simulink model "Custom_mod"  (R2021a)
settings: configuration reference "AION_IDS_Speedgoat" (kept outside this file)
undefined symbols (not defined in the file): EPSILON
libraries: simulink x1
Description:
  | 自定义取模
settings Model: DataDictionary=Custom_Mod.sldd  Creator=xinrui  LastModifiedBy=Administrator
settings ConfigSetRef: SourceName=AION_IDS_Speedgoat

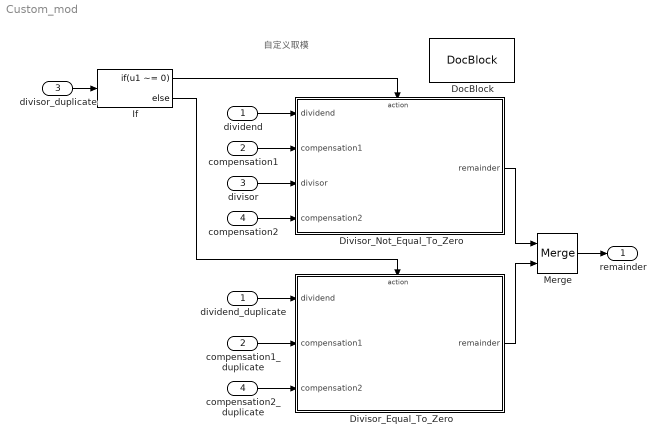
== system Custom_mod ==
  note: 自定义取模
  dividend : Inport  Description=被除数（待取模的数），实数，无量纲。  OutDataTypeStr=double  PortDimensions=1
  compensation1 : Inport  Description=用于调整取模前数值范围的补偿值1，实数，无量纲。  Port=2  OutDataTypeStr=double  PortDimensions=1
  divisor : Inport  Description=除数，实数，无量纲。  Port=3  OutDataTypeStr=double  PortDimensions=1
  compensation2 : Inport  Description=用于调整取模后数值范围的补偿值2，实数，无量纲。  Port=4  OutDataTypeStr=double  PortDimensions=1
  Divisor_Equal_To_Zero : Subsystem  Description=被除数等于0时直接输出被除数变换数值范围的结果。  TreatAsAtomicUnit=on
  Divisor_Not_Equal_To_Zero : Subsystem  Description=被除数不等于0时可依照公式计算余数，输出变换数值范围后的结果。  TreatAsAtomicUnit=on
  DocBlock : simulink/Model-Wide Utilities/DocBlock  DocumentType=HTML  mask(DocBlock){}
      mask Display:
      | plot([.8 0 0 1 1 .8 .8 1],[1 1 0 0 .8 1 .8 .8]);
      | text(.5,.6,'CHANGELOG','horizontalalignment','center');
      | text(.95,.05,get_param(gcb,'DocumentType'),'verticalalignment','bottom','horizontalalignment','right');
  If : If  IfExpression=u1 ~= 0
  Merge : Merge
  compensation1_duplicate : InportShadow  Description=用于调整取模前数值范围的补偿值1，实数，无量纲。  Port=2  OutDataTypeStr=double  PortDimensions=1
  compensation2_duplicate : InportShadow  Description=用于调整取模后数值范围的补偿值2，实数，无量纲。  Port=4  OutDataTypeStr=double  PortDimensions=1
  dividend_duplicate : InportShadow  Description=被除数（待取模的数），实数，无量纲。  OutDataTypeStr=double  PortDimensions=1
  divisor_duplicate : InportShadow  Description=除数，实数，无量纲。  Port=3  OutDataTypeStr=double  PortDimensions=1
  remainder : Outport  Description=余数，实数，无量纲。
  wires:
  dividend/1 -> Divisor_Not_Equal_To_Zero/1(dividend)
  compensation1/1 -> Divisor_Not_Equal_To_Zero/2(compensation1)
  divisor/1 -> Divisor_Not_Equal_To_Zero/3(divisor)
  compensation2/1 -> Divisor_Not_Equal_To_Zero/4(compensation2)
  divisor_duplicate/1 -> If/1
  If/1 -> Divisor_Not_Equal_To_Zero/Action
  Divisor_Not_Equal_To_Zero/1(remainder) -> Merge/1
  Divisor_Equal_To_Zero/1(remainder) -> Merge/2
  Merge/1 -> remainder/1
  compensation1_duplicate/1 -> Divisor_Equal_To_Zero/2(compensation1)
  compensation2_duplicate/1 -> Divisor_Equal_To_Zero/3(compensation2)
  dividend_duplicate/1 -> Divisor_Equal_To_Zero/1(dividend)
  If/2 -> Divisor_Equal_To_Zero/Action

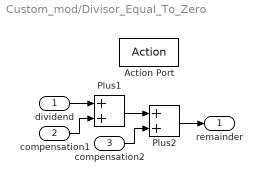
== system Custom_mod/Divisor_Equal_To_Zero ==
  dividend : Inport  Description=被除数（待取模的数），实数，无量纲。  OutDataTypeStr=double  PortDimensions=1
  compensation1 : Inport  Description=用于调整取模前数值范围的补偿值1，实数，无量纲。  Port=2  OutDataTypeStr=double  PortDimensions=1
  compensation2 : Inport  Description=用于调整取模后数值范围的补偿值2，实数，无量纲。  Port=3  OutDataTypeStr=double  PortDimensions=1
  Action Port : ActionPort  ActionPortLabel=else
  Plus1 : Sum  Description=将原始值通过补偿值1调整到指定数值范围区间。
  Plus2 : Sum  Description=将计算结果通过补偿值2调整到指定数值范围区间。
  remainder : Outport  Description=余数，实数，无量纲。
  wires:
  dividend/1 -> Plus1/1
  Plus2/1 -> remainder/1
  compensation2/1 -> Plus2/2
  Plus1/1 -> Plus2/1
  compensation1/1 -> Plus1/2

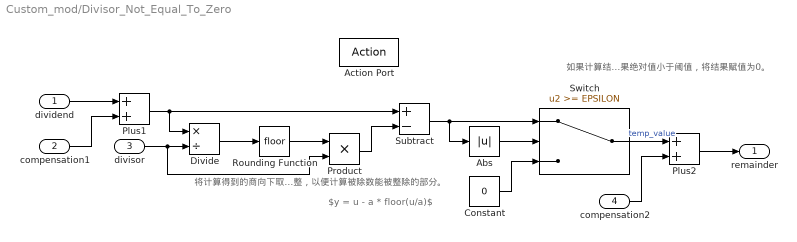
== system Custom_mod/Divisor_Not_Equal_To_Zero ==
  note: $y = u - a * floor(u/a)$
  note: 如果计算结果绝对值小于阈值，将结果赋值为0。
  note: 将计算得到的商向下取整，以便计算被除数能被整除的部分。
  dividend : Inport  Description=被除数（待取模的数），实数，无量纲。  OutDataTypeStr=double  PortDimensions=1
  compensation1 : Inport  Description=用于调整取模前数值范围的补偿值1，实数，无量纲。  Port=2  OutDataTypeStr=double  PortDimensions=1
  divisor : Inport  Description=除数，实数，无量纲。  Port=3  OutDataTypeStr=double  PortDimensions=1
  compensation2 : Inport  Description=用于调整取模后数值范围的补偿值2，实数，无量纲。  Port=4  OutDataTypeStr=double  PortDimensions=1
  Action Port : ActionPort  ActionPortLabel=if(u1 ~= 0)
  Abs : Abs
  Constant : Constant  Value=0  OutDataTypeStr=double  SampleTime=-1
  Divide : Product  Description=求被除数除以除数的商。  Inputs=*/
  Plus1 : Sum  Description=将原始值通过补偿值1调整到指定数值范围区间。
  Plus2 : Sum  Description=将计算结果通过补偿值2调整到指定数值范围区间。
  Product : Product  Description=将除数与整数形式的商相乘得到被除数能被整除部分
  Rounding Function : Rounding  Description=将计算得到的商向下取整，以便计算被除数能被整除的部分。
  Subtract : Sum  Description=将被除数减去能被整除部分，得到余数。  Inputs=+-
  Switch : Switch  Description=如果计算结果绝对值小于阈值，将结果赋值为0。  Threshold=EPSILON
  remainder : Outport  Description=余数，实数，无量纲。
  wires:
  Constant/1 -> Switch/3
  compensation2/1 -> Plus2/2
  Rounding Function/1 -> Product/1
  Plus2/1 -> remainder/1
  Divide/1 -> Rounding Function/1
  dividend/1 -> Plus1/1
  compensation1/1 -> Plus1/2
  Abs/1 -> Switch/2
  Switch/1 -> Plus2/1  "temp_value"
  Plus1/1 -> Subtract/1, Divide/1
  Product/1 -> Subtract/2
  divisor/1 -> Divide/2, Product/2
  Subtract/1 -> Switch/1, Abs/1
